simulink model "Two_stage_rectified_echo_detector"  (R2015a)
settings: Solver=ode23t  StartTime=0.0  StopTime=1  RelTol=1e-3
libraries: fl_lib x17, nesl_utility x6, elec_lib x5
settings Model: Creator=saifur  LastModifiedBy=saifur

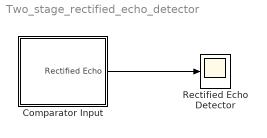
== system Two_stage_rectified_echo_detector ==
  Comparator Input : Subsystem
  Rectified Echo Detector : Scope
      settings: TimeRange=0.03899999999380732  YMin=-3.5  YMax=3.5
  wires:
  Comparator Input/1(Rectified Echo) -> Rectified Echo Detector/1

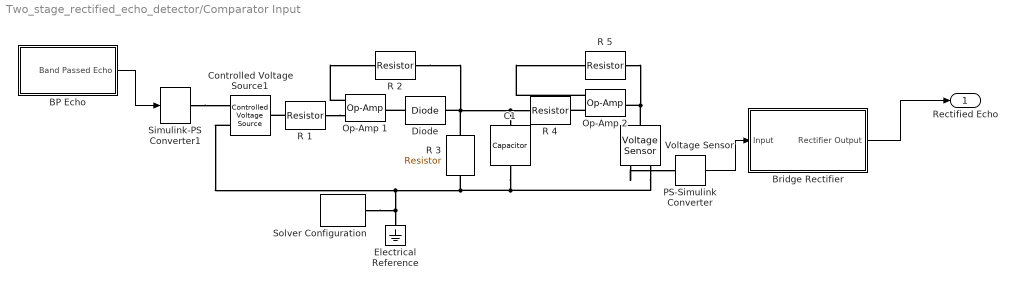
== system Two_stage_rectified_echo_detector/Comparator Input ==
  BP Echo : Subsystem
  "Bridge Rectifier " : Subsystem
  C1 : fl_lib/Electrical/Electrical Elements/Capacitor  c=1e-6 F  r=1e-6 Ohm  g=0 1/Ohm  i_specify=off  i_priority=High  i=0 A  v_specify=off  v_priority=High  v=0 V  vc_specify=off  vc_priority=High  vc=0 V
  Controlled Voltage Source1 : fl_lib/Electrical/Electrical Sources/Controlled Voltage Source
  Diode : fl_lib/Electrical/Electrical Elements/Diode  Vf=0.6 V  Ron=0.3 Ohm  Goff=1e-8 1/Ohm  i_specify=off  i_priority=High  i=0 A  v_specify=off  v_priority=High  v=0 V
  Electrical Reference : fl_lib/Electrical/Electrical Elements/Electrical Reference
  Op-Amp 1 : fl_lib/Electrical/Electrical Elements/Op-Amp  outI_specify=off  outI_priority=High  outI=0 A
  Op-Amp 2 : fl_lib/Electrical/Electrical Elements/Op-Amp  outI_specify=off  outI_priority=High  outI=0 A
  PS-Simulink Converter : nesl_utility/PS-Simulink Converter  PhysicalDomain=network_engine_domain  SubClassName=ps_output  LeftPortType=input  RightPortType=output  PseudoPeriodic=off  Frequencies=[]  Unit=1  AffineConversion=off
  R 1 : fl_lib/Electrical/Electrical Elements/Resistor  R=1 Ohm  i_specify=off  i_priority=High  i=0 A  v_specify=off  v_priority=High  v=0 V
  R 2 : elec_lib/Passive Devices/Resistor  R=1 Ohm  noise_mode=0  Tdevice=25 C  sample_time=0.001 s  repeatability=1  auto_seed=3499211588  user_seed=0
  R 3 : elec_lib/Passive Devices/Resistor  R=1 Ohm  noise_mode=0  Tdevice=25 C  sample_time=0.001 s  repeatability=1  auto_seed=3890346746  user_seed=0
  R 4 : elec_lib/Passive Devices/Resistor  R=1 Ohm  noise_mode=0  Tdevice=25 C  sample_time=0.001 s  repeatability=1  auto_seed=545404223  user_seed=0
  R 5 : elec_lib/Passive Devices/Resistor  R=1 Ohm  noise_mode=0  Tdevice=25 C  sample_time=0.001 s  repeatability=1  auto_seed=3922919431  user_seed=0
  Simulink-PS Converter1 : nesl_utility/Simulink-PS Converter  PhysicalDomain=network_engine_domain  SubClassName=ps_input  LeftPortType=input  RightPortType=output  PseudoPeriodic=off  Frequencies=[]  NoiseDistribution=none  NoiseParameters=[]  Unit=V  AffineConversion=off  InputFiltering=off  SimscapeFilterOrder=1  InputFilterTimeConstant=0.001  UdotUserProvided=1
  Solver Configuration : nesl_utility/Solver Configuration  PhysicalDomain=network_engine_domain  SubClassName=solver  LeftPortType=input  RightPortType=generic  Accelerate=off  Tones=[]  Harmonics=[]  SimulateNoise=off  Profile=off  UseLocalSampling=off  EnableSwitchedLinearOptims=on  FrequencyDomain=off  UseCCode=off  RelTol=0.001  AbsTol=1e-06  MinStep=1e-09  ToWorkspace=off  RevertToSquareIcSolve=off  NumHomotopyIterations=100  DoDC=on  ResidualTolerance=1e-09  UseLocalSolver=off  LocalSolverChoice=NE_BACKWARD_EULER_ADVANCER  LocalSolverSampleTime=0.001  DoFixedCost=off  MaxNonlinIter=3  MaxModeIter=2  LinearAlgebra=Sparse  DelaysMemoryBudget=1024  AutomaticFiltering=on  FilteringTimeConstant=0.001
  Voltage Sensor : fl_lib/Electrical/Electrical Sensors/Voltage Sensor
  Rectified Echo : Outport
  wires:
  "Bridge Rectifier "/1(Rectifier Output) -> Rectified Echo/1
  PS-Simulink Converter/1 -> "Bridge Rectifier "/1(Input)
  BP Echo/1("Band Passed Echo ") -> Simulink-PS Converter1/1
  connections:
  R 1/RConn1 -- Op-Amp 1/LConn1
  R 5/RConn1 -- Voltage Sensor/LConn1 -- Op-Amp 2/RConn1
  Voltage Sensor/RConn1 -- PS-Simulink Converter/LConn1
  Simulink-PS Converter1/RConn1 -- Controlled Voltage Source1/RConn1
  C1/RConn1 -- Voltage Sensor/RConn2 -- Solver Configuration/RConn1 -- Electrical Reference/LConn1 -- Controlled Voltage Source1/RConn2 -- R 3/RConn1
  Op-Amp 2/LConn2 -- R 5/LConn1
  R 1/LConn1 -- Controlled Voltage Source1/LConn1
  R 2/RConn1 -- R 4/LConn1 -- C1/LConn1 -- R 3/LConn1 -- Diode/RConn1
  Op-Amp 2/LConn1 -- R 4/RConn1
  Diode/LConn1 -- Op-Amp 1/RConn1
  Op-Amp 1/LConn2 -- R 2/LConn1

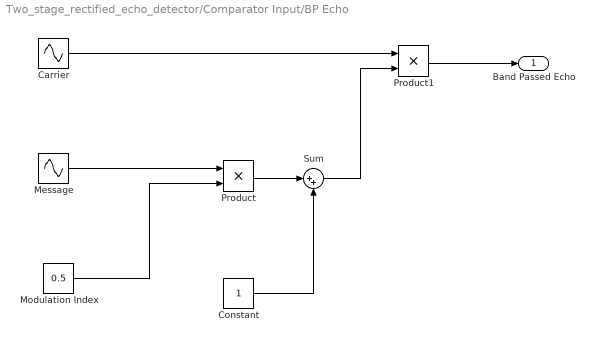
== system Two_stage_rectified_echo_detector/Comparator Input/BP Echo ==
  Carrier : Sin  Frequency=2*pi*100  SampleTime=1/5000
  Constant : Constant
  Message : Sin  Amplitude=5  Frequency=2*pi*10  SampleTime=1/5000
  Modulation Index : Constant  Value=0.5
  Product : Product
  Product1 : Product
  Sum : Sum  Inputs=|++
  "Band Passed Echo " : Outport
  wires:
  Product/1 -> Sum/1
  Modulation Index/1 -> Product/2
  Message/1 -> Product/1
  Constant/1 -> Sum/2
  Carrier/1 -> Product1/1
  Sum/1 -> Product1/2
  Product1/1 -> "Band Passed Echo "/1

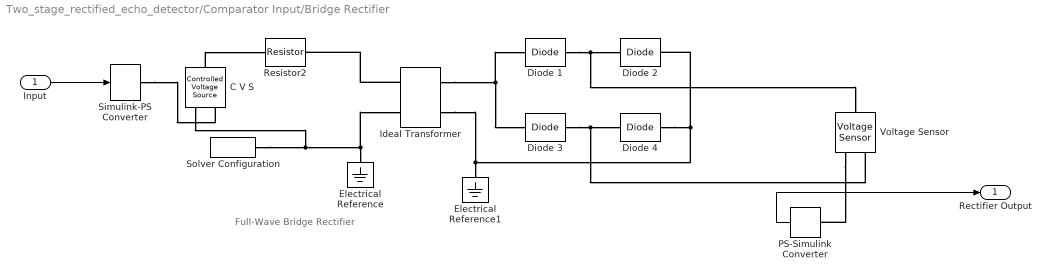
== system Two_stage_rectified_echo_detector/Comparator Input/Bridge Rectifier  ==
  note: Full-Wave Bridge Rectifier
  Input : Inport
  C V S : fl_lib/Electrical/Electrical Sources/Controlled Voltage Source
  Diode 1 : fl_lib/Electrical/Electrical Elements/Diode  Vf=0.0001 V  Ron=0.002 Ohm  Goff=1e-08 1/Ohm  i_specify=off  i_priority=High  i=0 A  v_specify=off  v_priority=High  v=0 V
  Diode 2 : fl_lib/Electrical/Electrical Elements/Diode  Vf=0.0002 V  Ron=0.002 Ohm  Goff=1e-08 1/Ohm  i_specify=off  i_priority=High  i=0 A  v_specify=off  v_priority=High  v=0 V
  Diode 3 : fl_lib/Electrical/Electrical Elements/Diode  Vf=0.002 V  Ron=0.003 Ohm  Goff=1e-08 1/Ohm  i_specify=off  i_priority=High  i=0 A  v_specify=off  v_priority=High  v=0 V
  Diode 4 : fl_lib/Electrical/Electrical Elements/Diode  Vf=0.002 V  Ron=0.002 Ohm  Goff=1e-08 1/Ohm  i_specify=off  i_priority=High  i=0 A  v_specify=off  v_priority=High  v=0 V
  Electrical Reference : fl_lib/Electrical/Electrical Elements/Electrical Reference
  Electrical Reference1 : fl_lib/Electrical/Electrical Elements/Electrical Reference
  Ideal Transformer : fl_lib/Electrical/Electrical Elements/Ideal Transformer  n=1  i1_specify=off  i1_priority=High  i1=0 A  v1_specify=off  v1_priority=High  v1=0 V  i2_specify=off  i2_priority=High  i2=0 A  v2_specify=off  v2_priority=High  v2=0 V
  PS-Simulink Converter : nesl_utility/PS-Simulink Converter  PhysicalDomain=network_engine_domain  SubClassName=ps_output  LeftPortType=input  RightPortType=output  PseudoPeriodic=off  Frequencies=[]  Unit=1  AffineConversion=off
  Resistor2 : elec_lib/Passive Devices/Resistor  R=10 Ohm  noise_mode=0  Tdevice=25 C  sample_time=0.001 s  repeatability=1  auto_seed=3499211588  user_seed=0
  Simulink-PS Converter : nesl_utility/Simulink-PS Converter  PhysicalDomain=network_engine_domain  SubClassName=ps_input  LeftPortType=input  RightPortType=output  PseudoPeriodic=off  Frequencies=[]  NoiseDistribution=none  NoiseParameters=[]  Unit=V  AffineConversion=off  InputFiltering=off  SimscapeFilterOrder=1  InputFilterTimeConstant=0.001  UdotUserProvided=1
  Solver Configuration : nesl_utility/Solver Configuration  PhysicalDomain=network_engine_domain  SubClassName=solver  LeftPortType=input  RightPortType=generic  Accelerate=off  Tones=[]  Harmonics=[]  SimulateNoise=off  Profile=off  UseLocalSampling=off  EnableSwitchedLinearOptims=on  FrequencyDomain=off  UseCCode=off  RelTol=0.001  AbsTol=1e-06  MinStep=1e-09  ToWorkspace=off  RevertToSquareIcSolve=off  NumHomotopyIterations=100  DoDC=off  ResidualTolerance=1e-9  UseLocalSolver=off  LocalSolverChoice=NE_BACKWARD_EULER_ADVANCER  LocalSolverSampleTime=.001  DoFixedCost=off  MaxNonlinIter=3  MaxModeIter=2  LinearAlgebra=Sparse  DelaysMemoryBudget=1024  AutomaticFiltering=on  FilteringTimeConstant=0.001
  Voltage Sensor : fl_lib/Electrical/Electrical Sensors/Voltage Sensor
  Rectifier Output : Outport
  wires:
  Input/1 -> Simulink-PS Converter/1
  PS-Simulink Converter/1 -> Rectifier Output/1
  connections:
  Simulink-PS Converter/RConn1 -- C V S/RConn1
  C V S/LConn1 -- Resistor2/LConn1
  Ideal Transformer/LConn1 -- Resistor2/RConn1
  Diode 3/LConn1 -- Diode 4/LConn1 -- Voltage Sensor/RConn2
  Ideal Transformer/RConn2 -- Diode 2/LConn1 -- Diode 4/RConn1 -- Electrical Reference1/LConn1
  Solver Configuration/RConn1 -- Ideal Transformer/LConn2 -- Electrical Reference/LConn1 -- C V S/RConn2
  Ideal Transformer/RConn1 -- Diode 3/RConn1 -- Diode 1/LConn1
  Diode 1/RConn1 -- Diode 2/RConn1 -- Voltage Sensor/LConn1
  Voltage Sensor/RConn1 -- PS-Simulink Converter/LConn1
